simulink model "nonlin_model_M8_slx"  (R2014a)
settings: Solver=ode113  SolverMode=SingleTasking  StartTime=0  StopTime=0.01  RelTol=1e-3  AbsTol=1e-3
settings Model: CovSFcnEnable=on  Creator=gladkikh  LastModifiedBy=User
settings SolverCC: ZeroCrossAlgorithm=Adaptive
settings DataIOCC: LimitDataPoints=off  SignalLoggingSaveFormat=ModelDataLogs  SignalLoggingName=sigsOut
settings OptimizationCC: BlockReduction=off  BooleanDataType=off  InlineParams=on  BufferReuse=off  ExpressionDepthLimit=2147483647  InitFltsAndDblsToZero=on  SimCompilerOptimization=off
settings DebuggingCC: AlgebraicLoopMsg=none  SaveWithParameterizedLinksMsg=none  UnderspecifiedInitializationDetection=Classic  SignalResolutionControl=TryResolveAllWithWarning  SolverPrmCheckMsg=none  MultiTaskDSMMsg=warning  MultiTaskCondExecSysMsg=none  FcnCallInpInsideContextMsg=UseLocalSettings  UnconnectedInputMsg=none  UnconnectedOutputMsg=none  UnconnectedLineMsg=none  FrameProcessingCompatibilityMsg=error  StateNameClashWarn=warning
settings HardwareCC: TargetBitPerLong=64  TargetBitPerPointer=64  TargetLongLongMode=on  TargetEndianess=LittleEndian  TargetWordSize=64  TargetHWDeviceType=MATLAB Host  ProdEqTarget=off
settings RTWCC: RTWCompilerOptimization=off
settings GRTTargetCC: TargetFcnLib=ansi_tfl_tmw.mat  CombineOutputUpdateFcns=off  GRTInterface=on

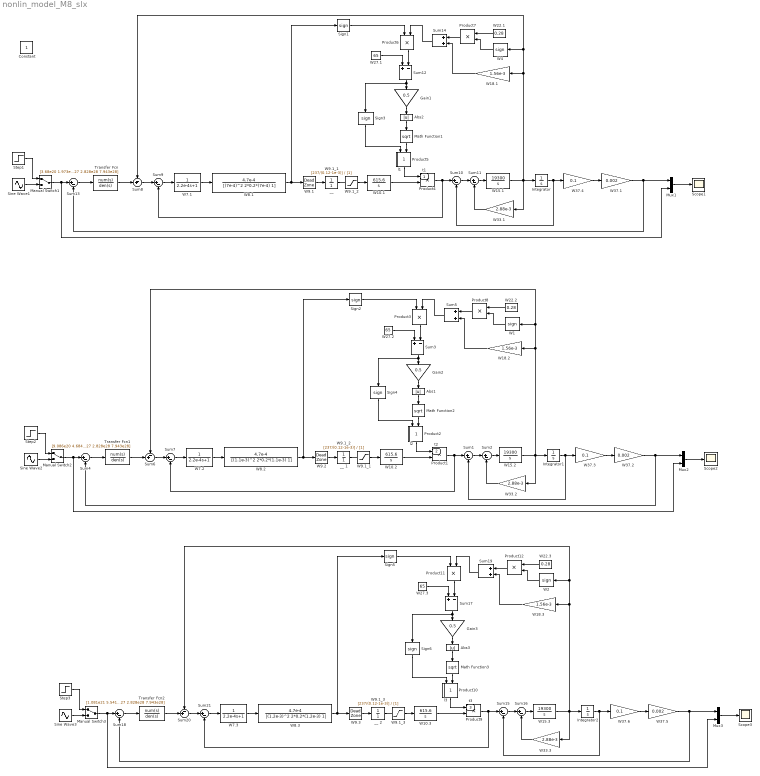
== system nonlin_model_M8_slx ==
  " W9.1_1" : TransferFcn  Numerator=[237/(0.12-1e-3)]  Denominator=[1]
  " W9.1_2" : TransferFcn  Numerator=[237/(0.12-1e-3)]  Denominator=[1]
  " W9.1_3" : TransferFcn  Numerator=[237/(0.12-1e-3)]  Denominator=[1]
  Abs1 : Abs  SaturateOnIntegerOverflow=on
  Abs2 : Abs  SaturateOnIntegerOverflow=on
  Abs3 : Abs  SaturateOnIntegerOverflow=on
  Gain1 : Gain  Gain=0.5  SaturateOnIntegerOverflow=on  OutDataTypeStr=Inherit: Same as input  ParamDataTypeStr=Inherit: Same as input
  Gain2 : Gain  Gain=0.5  SaturateOnIntegerOverflow=on  OutDataTypeStr=Inherit: Same as input  ParamDataTypeStr=Inherit: Same as input
  Gain3 : Gain  Gain=0.5  SaturateOnIntegerOverflow=on  OutDataTypeStr=Inherit: Same as input  ParamDataTypeStr=Inherit: Same as input
  Integrator : Integrator
  Integrator1 : Integrator
  Integrator2 : Integrator
  Manual Switch1 : ManualSwitch
  Manual Switch2 : ManualSwitch
  Manual Switch3 : ManualSwitch
  Math Function1 : Math  Operator=sqrt  SaturateOnIntegerOverflow=on
  Math Function2 : Math  Operator=sqrt  SaturateOnIntegerOverflow=on
  Math Function3 : Math  Operator=sqrt  SaturateOnIntegerOverflow=on
  Mux1 : Mux  Inputs=2
  Mux2 : Mux  Inputs=2
  Mux3 : Mux  Inputs=2
  Product{1..12} (12 alike) : Product  SaturateOnIntegerOverflow=on  InputSameDT=on  OutDataTypeStr=Inherit: Same as first input
  Scope1 : Scope
      settings: YMin=1  YMax=1.04
  Scope2 : Scope
      settings: YMin=1  YMax=1.04
  Scope3 : Scope
      settings: YMin=1  YMax=1.04  SaveName=ScopeData2
  Sign{1..6} (6 alike) : Signum
  Sine Wave1 : Sin  Frequency=1000  SampleTime=0
  Sine Wave2 : Sin  Frequency=1000  SampleTime=0
  Sine Wave3 : Sin  Frequency=1000  SampleTime=0
  Step1 : Step  Time=0  SampleTime=0
  Step2 : Step  Time=0  SampleTime=0
  Step3 : Step  Time=0  SampleTime=0
  Sum{1..2,4,7,9..11,13,15..16,18,21} (12 alike) : Sum  Inputs=|+-
  Sum12 : Sum  Inputs=+-  SaturateOnIntegerOverflow=on  InputSameDT=on  OutDataTypeStr=Inherit: Same as first input
  Sum14 : Sum  SaturateOnIntegerOverflow=on  InputSameDT=on  OutDataTypeStr=Inherit: Same as first input
  Sum17 : Sum  Inputs=+-  SaturateOnIntegerOverflow=on  InputSameDT=on  OutDataTypeStr=Inherit: Same as first input
  Sum19 : Sum  SaturateOnIntegerOverflow=on  InputSameDT=on  OutDataTypeStr=Inherit: Same as first input
  Sum20 : Sum  Inputs=-+|
  Sum3 : Sum  Inputs=+-  SaturateOnIntegerOverflow=on  InputSameDT=on  OutDataTypeStr=Inherit: Same as first input
  Sum5 : Sum  SaturateOnIntegerOverflow=on  InputSameDT=on  OutDataTypeStr=Inherit: Same as first input
  Sum6 : Sum  Inputs=-+|
  Sum8 : Sum  Inputs=-+|
  Transfer Fcn : TransferFcn  Numerator=[3.68e20 1.973e24 2.18e27 3.893e30 8.987e32 1.298e35 1.447e37 2.854e36]  Denominator=[1 1.539e06 8.565e11 2.152e17 2.439e22 1.001e27 2.828e28 7.943e28]
  Transfer Fcn1 : TransferFcn  Numerator=[9.086e20 4.684e24 3.376e27 4.11e30 9.247e32 1.317e35 1.447e37 2.854e36]  Denominator=[1 1.539e06 8.565e11 2.152e17 2.439e22 1.001e27 2.828e28 7.943e28]
  Transfer Fcn2 : TransferFcn  Numerator=[1.081e21 5.541e24 3.718e27 4.17e30 9.317e32 1.321e35 1.447e37 2.854e36]  Denominator=[1 1.539e06 8.565e11 2.152e17 2.439e22 1.001e27 2.828e28 7.943e28]
  W1 : Signum
  W10.1 : TransferFcn  Numerator=[615.6]  Denominator=[1 0]
  W10.2 : TransferFcn  Numerator=[615.6]  Denominator=[1 0]
  W10.3 : TransferFcn  Numerator=[615.6]  Denominator=[1 0]
  W15.1 : TransferFcn  Numerator=[19300]  Denominator=[1 0]
  W15.2 : TransferFcn  Numerator=[19300]  Denominator=[1 0]
  W15.3 : TransferFcn  Numerator=[19300]  Denominator=[1 0]
  W18.1 : Gain  Gain=1.56e-3  SaturateOnIntegerOverflow=on  OutDataTypeStr=Inherit: Same as input  ParamDataTypeStr=Inherit: Same as input
  W18.2 : Gain  Gain=1.56e-3  SaturateOnIntegerOverflow=on  OutDataTypeStr=Inherit: Same as input  ParamDataTypeStr=Inherit: Same as input
  W18.3 : Gain  Gain=1.56e-3  SaturateOnIntegerOverflow=on  OutDataTypeStr=Inherit: Same as input  ParamDataTypeStr=Inherit: Same as input
  W2 : Signum
  W22.1 : Constant  Value=0.28
  W22.2 : Constant  Value=0.28
  W22.3 : Constant  Value=0.28
  W27.1 : Constant  Value=65
  W27.2 : Constant  Value=65
  W27.3 : Constant  Value=65
  W33.1 : Gain  Gain=2.88e-3  SaturateOnIntegerOverflow=on  OutDataTypeStr=Inherit: Same as input  ParamDataTypeStr=Inherit: Same as input
  W33.2 : Gain  Gain=2.88e-3  SaturateOnIntegerOverflow=on  OutDataTypeStr=Inherit: Same as input  ParamDataTypeStr=Inherit: Same as input
  W33.3 : Gain  Gain=2.88e-3  SaturateOnIntegerOverflow=on  OutDataTypeStr=Inherit: Same as input  ParamDataTypeStr=Inherit: Same as input
  W37.1 : Gain  Gain=0.002
  W37.2 : Gain  Gain=0.002
  W37.3 : Gain  Gain=0.1
  W37.4 : Gain  Gain=0.1
  W37.5 : Gain  Gain=0.002
  W37.6 : Gain  Gain=0.1
  W4 : Signum
  W7.1 : TransferFcn  Denominator=[2.2e-4 1]
  W7.2 : TransferFcn  Denominator=[2.2e-4 1]
  W7.3 : TransferFcn  Denominator=[2.2e-4 1]
  W8.1 : TransferFcn  Numerator=[4.7e-4]  Denominator=[(7e-4)^2 2*0.2*(7e-4) 1]
  W8.2 : TransferFcn  Numerator=[4.7e-4]  Denominator=[(1.1e-3)^2 2*0.2*(1.1e-3) 1]
  W8.3 : TransferFcn  Numerator=[4.7e-4]  Denominator=[(1.2e-3)^2 2*0.2*(1.2e-3) 1]
  W9.1 : DeadZone  LowerValue=-1e-3  UpperValue=1e-3  SaturateOnIntegerOverflow=on
  W9.1_1 : Saturate  UpperLimit=237  LowerLimit=-237
  W9.1_2 : Saturate  UpperLimit=237  LowerLimit=-237
  W9.1_3 : Saturate  UpperLimit=237  LowerLimit=-237
  W9.2 : DeadZone  LowerValue=-1e-3  UpperValue=1e-3  SaturateOnIntegerOverflow=on
  W9.3 : DeadZone  LowerValue=-1e-3  UpperValue=1e-3  SaturateOnIntegerOverflow=on
  "__ " : TransferFcn  Numerator=1  Denominator=[1]
  __ 1 : TransferFcn  Numerator=1  Denominator=[1]
  __ 2 : TransferFcn  Numerator=1  Denominator=[1]
  l1 : Constant
  l2 : Constant
  l3 : Constant
  t1 : Outport
  t2 : Outport  Port=2
  t3 : Outport  Port=3
  Constant : Constant  IOType=siggen
  wires:
  Manual Switch1/1 -> Sum13/1, Mux1/2
  Step1/1 -> Manual Switch1/1
  Sum9/1 -> W7.1/1
  W15.1/1 -> Integrator/1, W33.1/1, W18.1/1, Sum8/1, W4/1
  Math Function1/1 -> Product5/2
  W8.1/1 -> Sign1/1, W9.1/1
  Gain1/1 -> Abs2/1
  Abs2/1 -> Math Function1/1
  Sum12/1 -> Gain1/1, Sign3/1
  W22.1/1 -> Product7/1
  W7.1/1 -> W8.1/1
  Product6/1 -> Sum12/2
  W27.1/1 -> Sum12/1
  Sine Wave1/1 -> Manual Switch1/2
  Mux1/1 -> Scope1/1
  W33.1/1 -> Sum11/2
  Sum11/1 -> W15.1/1
  Sum10/1 -> Sum11/1
  Sum8/1 -> Sum9/1
  Sum14/1 -> Product6/2
  Product7/1 -> Sum14/1
  W18.1/1 -> Sum14/2
  Sum13/1 -> Transfer Fcn/1
  Product4/1 -> Sum10/1, Sum9/2
  W10.1/1 -> Product4/2
  Sign1/1 -> Product6/1
  Sign3/1 -> Product5/1
  W4/1 -> Product7/2
  Transfer Fcn/1 -> Sum8/2
  l1/1 -> Product4/1
  Product5/1 -> t1/1
  Integrator/1 -> W37.4/1, Sum10/2
  W37.1/1 -> Mux1/1, Sum13/2
  W9.1/1 -> "__ "/1
  "__ "/1 -> W10.1/1
  " W9.1_1"/1 -> " W9.1_1"/1
  W9.1_2/1 -> W9.1_2/1
  W37.4/1 -> W37.1/1
  Manual Switch2/1 -> Sum4/1, Mux2/2
  Step2/1 -> Manual Switch2/1
  Sum7/1 -> W7.2/1
  W15.2/1 -> Integrator1/1, W33.2/1, W18.2/1, Sum6/1, W1/1
  Math Function2/1 -> Product2/2
  W8.2/1 -> Sign2/1, W9.2/1
  Gain2/1 -> Abs1/1
  Abs1/1 -> Math Function2/1
  Sum3/1 -> Gain2/1, Sign4/1
  W22.2/1 -> Product8/1
  W7.2/1 -> W8.2/1
  Product3/1 -> Sum3/2
  W27.2/1 -> Sum3/1
  Sine Wave2/1 -> Manual Switch2/2
  Mux2/1 -> Scope2/1
  W33.2/1 -> Sum2/2
  Sum2/1 -> W15.2/1
  Sum1/1 -> Sum2/1
  Sum6/1 -> Sum7/1
  Sum5/1 -> Product3/2
  Product8/1 -> Sum5/1
  W18.2/1 -> Sum5/2
  Sum4/1 -> Transfer Fcn1/1
  Product1/1 -> Sum1/1, Sum7/2
  W10.2/1 -> Product1/2
  Sign2/1 -> Product3/1
  Sign4/1 -> Product2/1
  W1/1 -> Product8/2
  Transfer Fcn1/1 -> Sum6/2
  l2/1 -> Product1/1
  Product2/1 -> t2/1
  Integrator1/1 -> W37.3/1, Sum1/2
  W37.2/1 -> Mux2/1, Sum4/2
  W9.2/1 -> __ 1/1
  __ 1/1 -> W10.2/1
  " W9.1_2"/1 -> " W9.1_2"/1
  W9.1_1/1 -> W9.1_1/1
  W37.3/1 -> W37.2/1
  Manual Switch3/1 -> Sum18/1, Mux3/2
  Step3/1 -> Manual Switch3/1
  Sum21/1 -> W7.3/1
  W15.3/1 -> Integrator2/1, W33.3/1, W18.3/1, Sum20/1, W2/1
  Math Function3/1 -> Product10/2
  W8.3/1 -> Sign5/1, W9.3/1
  Gain3/1 -> Abs3/1
  Abs3/1 -> Math Function3/1
  Sum17/1 -> Gain3/1, Sign6/1
  W22.3/1 -> Product12/1
  W7.3/1 -> W8.3/1
  Product11/1 -> Sum17/2
  W27.3/1 -> Sum17/1
  Sine Wave3/1 -> Manual Switch3/2
  Mux3/1 -> Scope3/1
  W33.3/1 -> Sum16/2
  Sum16/1 -> W15.3/1
  Sum15/1 -> Sum16/1
  Sum20/1 -> Sum21/1
  Sum19/1 -> Product11/2
  Product12/1 -> Sum19/1
  W18.3/1 -> Sum19/2
  Sum18/1 -> Transfer Fcn2/1
  Product9/1 -> Sum15/1, Sum21/2
  W10.3/1 -> Product9/2
  Sign5/1 -> Product11/1
  Sign6/1 -> Product10/1
  W2/1 -> Product12/2
  Transfer Fcn2/1 -> Sum20/2
  l3/1 -> Product9/1
  Product10/1 -> t3/1
  Integrator2/1 -> W37.6/1, Sum15/2
  W37.5/1 -> Mux3/1, Sum18/2
  W9.3/1 -> __ 2/1
  __ 2/1 -> W10.3/1
  " W9.1_3"/1 -> " W9.1_3"/1
  W9.1_3/1 -> W9.1_3/1
  W37.6/1 -> W37.5/1
